simulink model "simu_MPC_deadtime"  (R2023b)
settings: Solver=VariableStepAuto  StartTime=0.0  StopTime=Tsim  RelTol=1e-3
values from neighbouring files (symbols this model uses):
  A = [A1 zeros(size(A1)); zeros(size(A2)) A2]    [MPC_MIMO.m]    (also in MPC_MIMO_deadtime.m; MPC_MIMO_quadprog.m)
  B = [B1 B2; B3 B4]    [MPC_MIMO.m]    (also in MPC_MIMO_deadtime.m; MPC_MIMO_quadprog.m)
  D = [D1 zeros(size(D1)); zeros(size(D2)) D2]    [MPC_MIMO.m]    (also in MPC_MIMO_deadtime.m; MPC_MIMO_quadprog.m)
  H = [H zeros(size(H)); zeros(size(H)) H]    [MPC_MIMO.m]    (also in MPC_MIMO_deadtime.m; MPC_MIMO_quadprog.m)
  KF = K*F    [MPC_MIMO.m]    (also in MPC_MIMO_deadtime.m)
  Kr = [sum(K(1, 1:2:2*N)), sum(K(1, 2:2:2*N)) ... (first row only)    [MPC_MIMO.m]    (also in MPC_MIMO_deadtime.m)
undefined symbols (not defined in the file or in its folder): dist, ref, Tdist
libraries: cstblocks x2
settings Model: Creator=sergio  LastModifiedBy=sergio

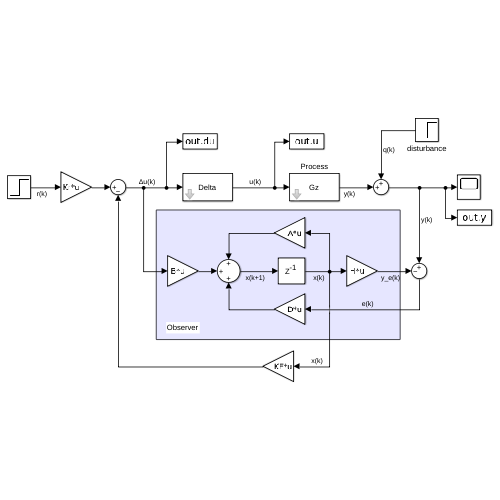
[thumbnail: Simulink's stored preview of the top-level diagram]
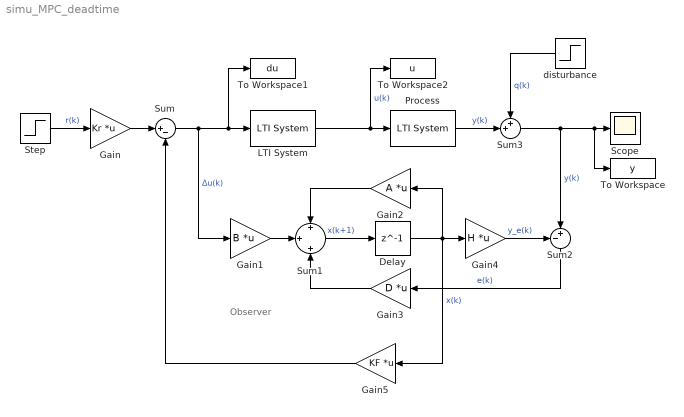
== system simu_MPC_deadtime ==
  note: Observer
  Delay : Delay  DelayLength=1
  Gain : Gain  Gain=Kr  Multiplication=Matrix(K*u)
  Gain1 : Gain  Gain=B  Multiplication=Matrix(K*u)
  Gain2 : Gain  Gain=A  Multiplication=Matrix(K*u)
  Gain3 : Gain  Gain=D  Multiplication=Matrix(K*u)
  Gain4 : Gain  Gain=H  Multiplication=Matrix(K*u)
  Gain5 : Gain  Gain=KF  Multiplication=Matrix(K*u)
  LTI System : cstblocks/LTI System  sys=Delta  IC=[]  PadeOrder=0
  Process : cstblocks/LTI System  sys=Gz  IC=[]  PadeOrder=0
  Scope : Scope
  Step : Step  Time=0  After=ref  SampleTime=0
  Sum : Sum  Inputs=|+-
  Sum1 : Sum  Inputs=+|+|+
  Sum2 : Sum  Inputs=-+|
  Sum3 : Sum  Inputs=++|
  To Workspace : ToWorkspace  VariableName=y  SampleTime=-1
  To Workspace1 : ToWorkspace  VariableName=du  SampleTime=-1
  To Workspace2 : ToWorkspace  VariableName=u  SampleTime=-1
  disturbance : Step  Time=Tdist  After=dist  SampleTime=0
  wires:
  Sum/1 -> Gain1/1, To Workspace1/1, LTI System/1  "Δu(k)"
  LTI System/1 -> To Workspace2/1, Process/1  "u(k)"
  Step/1 -> Gain/1  "r(k)"
  Gain/1 -> Sum/1
  Gain1/1 -> Sum1/2
  Gain4/1 -> Sum2/1  "y_e(k)"
  Delay/1 -> Gain2/1, Gain5/1, Gain4/1  "x(k)"
  Sum1/1 -> Delay/1  "x(k+1)"
  Sum2/1 -> Gain3/1  "e(k)"
  Gain2/1 -> Sum1/1
  Gain3/1 -> Sum1/3
  Gain5/1 -> Sum/2
  Process/1 -> Sum3/2  "y(k)"
  Sum3/1 -> Sum2/2, To Workspace/1, Scope/1  "y(k)"
  disturbance/1 -> Sum3/1  "q(k)"
